simulink model "Guidance_loop"  (R2025b)
settings: Solver=VariableStepAuto  StartTime=0.0  StopTime=10.0  RelTol=1e-3
settings Model: Creator=samue  LastModifiedBy=samue

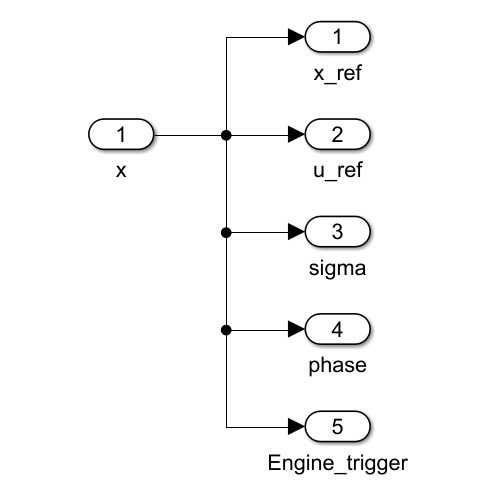
[thumbnail: Simulink's stored preview of the top-level diagram]
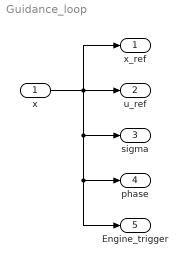
== system Guidance_loop ==
  x : Inport
  x_ref : Outport
  u_ref : Outport  Port=2
  sigma : Outport  Port=3
  phase : Outport  Port=4
  Engine_trigger : Outport  Port=5
  wires:
  x/1 -> x_ref/1, sigma/1, phase/1, Engine_trigger/1, u_ref/1
